simulink subsystem "control_allocation"  (R2023a)
settings: Solver=VariableStepAuto  StartTime=0.0  StopTime=10.0  RelTol=1e-3
undefined symbols (not defined in the file or in its folder): Ginv, k_loss, kF, kM, max_ang_vel_motor, param
libraries: aerolibatmos2 x1
settings Model: Creator=raduserseniuc  LastModifiedBy=raduserseniuc

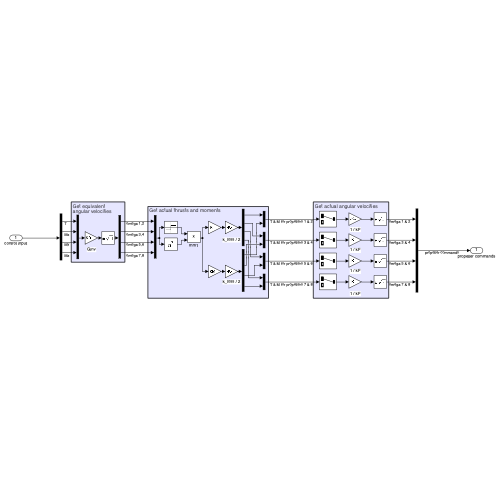
[thumbnail: Simulink's stored preview of the top-level diagram]
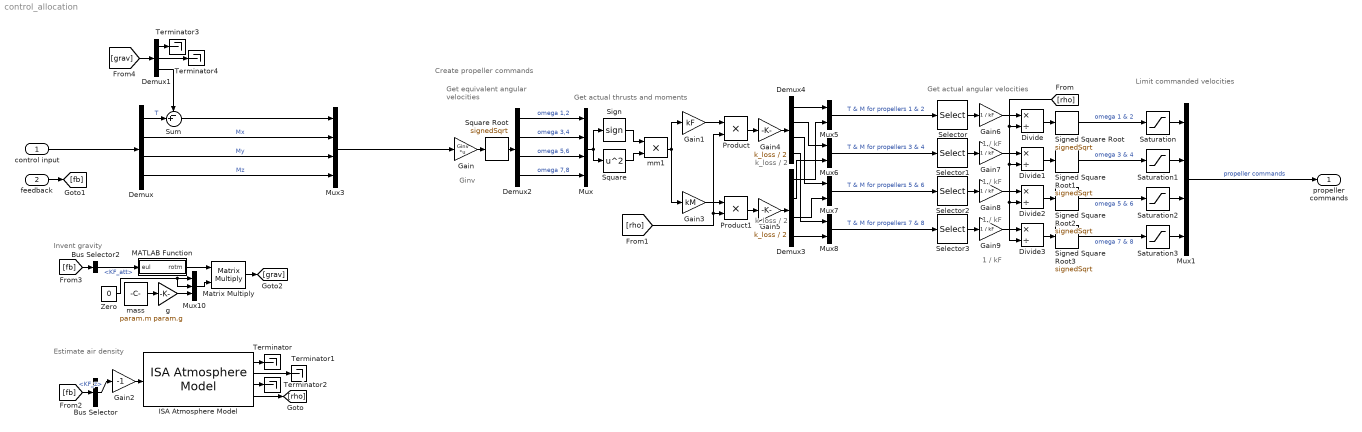
== system control_allocation ==
  note: Create propeller commands
  note: Limit
      | commanded
      | velocities
  note: Estimate air density
  note: 1 / kF
  note: k_loss / 2
  note: 1 / kF
  note: Get actual angular velocities
  note: Ginv
  note: Get equivalent
      | angular velocities
  note: 1 / kF
  note: Get actual thrusts and moments
  note: 1 / kF
  note: k_loss / 2
  note: Invent gravity
  control input : Inport
  feedback : Inport  Port=2
  Bus Selector : BusSelector  OutputSignals=x_filt.KF_pos.KF_z
  Bus Selector2 : BusSelector  OutputSignals=x_filt.KF_att
  Demux{,2..4} (4 alike) : Demux
  Demux1 : Demux  Outputs=3
  Divide{,1..3} (4 alike) : Product  Inputs=*/  RndMeth=Zero  SaturateOnIntegerOverflow=on
  Gain : Gain  Gain=Ginv  Multiplication=Matrix(K*u)
  Gain1 : Gain  Gain=kF
  Gain2 : Gain  Gain=-1
  Gain3 : Gain  Gain=kM
  Gain4 : Gain  Gain=k_loss / 2
  Gain5 : Gain  Gain=k_loss / 2
  Gain{6..9} (4 alike) : Gain  Gain=1 / kF
  ISA Atmosphere Model : aerolibatmos2/ISA Atmosphere Model  custom=off  g=9.80665  gamma=1.4  R=287.0531  L=0.0065  h_trop=11000  h_strat=20000  rho0=1.225  P0=101325  T0=288.15  h0=0
  MATLAB Function : MATLAB Function  TreatAsAtomicUnit=on
  Matrix Multiply : Product  Inputs=**  Multiplication=Matrix(*)
  Mux : Mux
  Mux1 : Mux
  Mux10 : Mux  Inputs=3
  Mux3 : Mux
  Mux{5..8} (4 alike) : Mux  Inputs=2
  Product : Product
  Product1 : Product
  Saturation{,1..3} (4 alike) : Saturate  UpperLimit=max_ang_vel_motor  LowerLimit=0
  Selector{,1..3} (4 alike) : Selector  InputPortWidth=2  IndexOptions=Index vector (dialog)  Indices=1  OutputSizes=1
  Sign : Signum
  Signed Square Root{,1..3} (4 alike) : Sqrt  Operator=signedSqrt
  Square : Math  Operator=square  SignedPower=on  RndMeth=Zero
  Square Root : Sqrt  Operator=signedSqrt
  Sum : Sum  Inputs=-+|
  Terminator{,1..4} (5 alike) : Terminator
  Zero : Constant  Value=0  OutDataTypeStr=Inherit: Inherit via back propagation
  g : Gain  Gain=param.g
  mass : Constant  Value=param.m
  mm1 : Product
  propeller commands : Outport
  wires:
  Gain8/1 -> Divide2/1
  Square/1 -> mm1/2
  Demux4/1 -> Mux5/1
  Gain/1 -> Square Root/1
  Selector1/1 -> Gain7/1
  Demux4/4 -> Mux8/1
  Gain3/1 -> Product1/1
  Mux/1 -> Square/1, Sign/1
  Demux4/3 -> Mux7/1
  Mux3/1 -> Gain/1
  Selector2/1 -> Gain8/1
  Mux6/1 -> Selector1/1  "T & M for propellers 3 & 4"
  Mux1/1 -> propeller commands/1  "propeller commands"
  Demux3/4 -> Mux8/2
  Gain7/1 -> Divide1/1
  Demux/4 -> Mux3/4  "Mz"
  Gain4/1 -> Demux4/1
  Gain9/1 -> Divide3/1
  Square Root/1 -> Demux2/1
  Signed Square Root2/1 -> Saturation2/1  "omega 5 & 6"
  Signed Square Root3/1 -> Saturation3/1  "omega 7 & 8"
  Demux/3 -> Mux3/3  "My"
  Selector/1 -> Gain6/1
  Gain1/1 -> Product/1
  Gain6/1 -> Divide/1
  Demux3/2 -> Mux6/2
  Demux3/1 -> Mux5/2
  Mux7/1 -> Selector2/1  "T & M for propellers 5 & 6"
  Signed Square Root1/1 -> Saturation1/1  "omega 3 & 4"
  Mux5/1 -> Selector/1  "T & M for propellers 1 & 2"
  Demux4/2 -> Mux6/1
  Selector3/1 -> Gain9/1
  Demux3/3 -> Mux7/2
  mm1/1 -> Gain3/1, Gain1/1
  Signed Square Root/1 -> Saturation/1  "omega 1 & 2"
  Gain5/1 -> Demux3/1
  control input/1 -> Demux/1
  Demux/2 -> Mux3/2  "Mx"
  Sign/1 -> mm1/1
  Mux8/1 -> Selector3/1  "T & M for propellers 7 & 8"
  Product/1 -> Gain4/1
  Product1/1 -> Gain5/1
  [rho] -> Divide/2, Divide1/2, Divide2/2, Divide3/2
  Divide/1 -> Signed Square Root/1
  Divide1/1 -> Signed Square Root1/1
  Divide2/1 -> Signed Square Root2/1
  Divide3/1 -> Signed Square Root3/1
  Gain2/1 -> ISA Atmosphere Model/1
  Demux2/1 -> Mux/1  "omega 1,2"
  Demux2/2 -> Mux/2  "omega 3,4"
  Demux2/3 -> Mux/3  "omega 5,6"
  Demux2/4 -> Mux/4  "omega 7,8"
  Saturation/1 -> Mux1/1
  Saturation1/1 -> Mux1/2
  Saturation2/1 -> Mux1/3
  Saturation3/1 -> Mux1/4
  ISA Atmosphere Model/1 -> Terminator/1
  ISA Atmosphere Model/2 -> Terminator1/1
  ISA Atmosphere Model/3 -> Terminator2/1
  [fb] -> Bus Selector/1
  Bus Selector/1 -> Gain2/1  "<KF_z>"
  ISA Atmosphere Model/4 -> [rho]
  [rho] -> Product1/2, Product/2
  [fb] -> Bus Selector2/1
  mass/1 -> g/1
  Mux10/1 -> Matrix Multiply/2
  Zero/1 -> Mux10/2, Mux10/1
  g/1 -> Mux10/3
  feedback/1 -> [fb]
  Bus Selector2/1 -> MATLAB Function/1(eul)  "<KF_att>"
  MATLAB Function/1(rotm) -> Matrix Multiply/1
  Matrix Multiply/1 -> [grav]
  [grav] -> Demux1/1
  Demux1/1 -> Terminator3/1
  Demux1/2 -> Terminator4/1
  Demux1/3 -> Sum/1
  Demux/1 -> Sum/2  "T"
  Sum/1 -> Mux3/1

== matlab function control_allocation/MATLAB Function ==
  data: eul input; rotm output
function rotm = fcn(eul)

rotm = eul2rotm(transpose(eul));
